simulink model "tankmodel_nonlinear_control101"  (R2025b)
settings: Solver=VariableStepAuto  StartTime=0.0  StopTime=300  RelTol=1e-3
undefined symbols (not defined in the file or in its folder): beta1rel, beta2rel, gamma1rel, gamma2rel
settings Model: Creator=barsr  LastModifiedBy=barsr
settings RTWCC: GPUComputeCapability=3.5

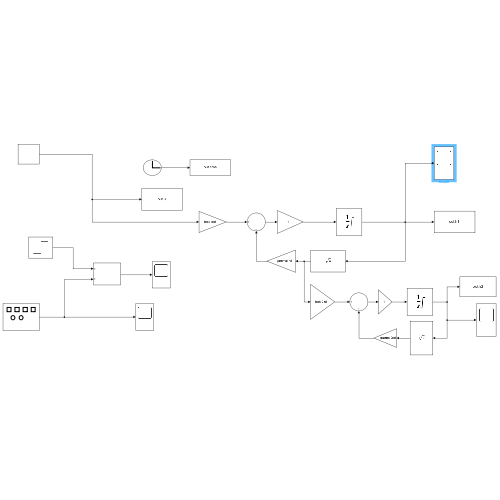
[thumbnail: Simulink's stored preview of the top-level diagram]
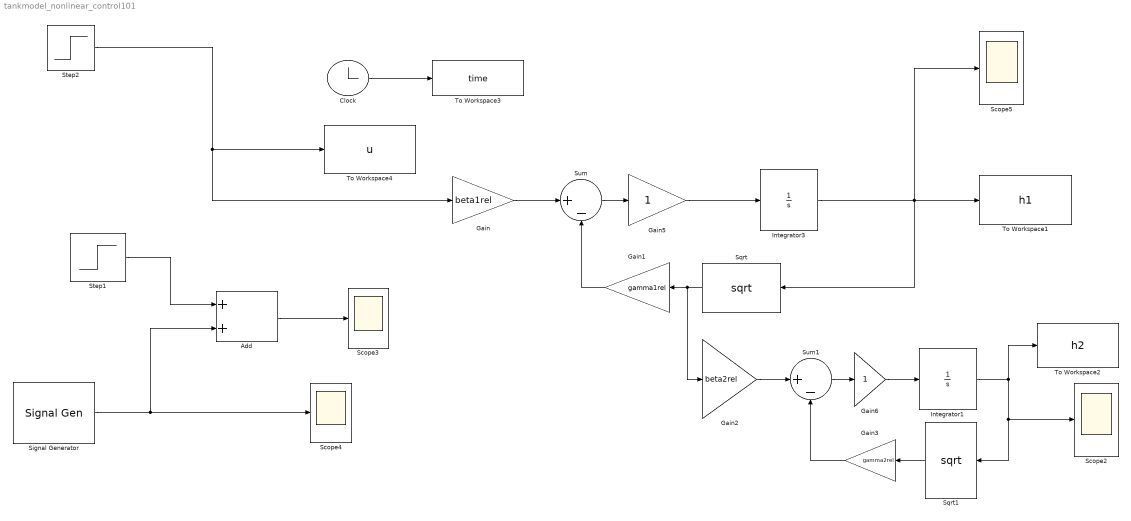
== system tankmodel_nonlinear_control101 ==
  Add : Sum
  Clock : Clock
  Gain : Gain  Gain=beta1rel
  Gain1 : Gain  Gain=gamma1rel
  Gain2 : Gain  Gain=beta2rel
  Gain3 : Gain  Gain=gamma2rel
  Gain5 : Gain
  Gain6 : Gain
  Integrator1 : Integrator  LimitOutput=on  UpperSaturationLimit=1  LowerSaturationLimit=0
  Integrator3 : Integrator  LimitOutput=on  UpperSaturationLimit=1  LowerSaturationLimit=0
  Scope{2..5} (4 alike) : Scope
      Scope2 settings: ActiveDisplayYMinimum=-0.53578092616151429  ActiveDisplayYMaximum=1.0409994632402184
      Scope3 settings: ActiveDisplayYMinimum=-1  ActiveDisplayYMaximum=1
      Scope4 settings: ActiveDisplayYMinimum=-1  ActiveDisplayYMaximum=1
      Scope5 settings: ActiveDisplayYMinimum=-0.01990953109028069  ActiveDisplayYMaximum=0.17918577981252626  DataLoggingVariableName=ScopeData2
  Signal Generator : SignalGenerator  WaveForm=square  Amplitude=0.05  Frequency=0.01  Units=rad/sec
  Sqrt : Sqrt
  Sqrt1 : Sqrt
  Step1 : Step  Time=0  After=0.25  SampleTime=0
  Step2 : Step  Time=0  After=0.25  SampleTime=0
  Sum : Sum  Inputs=|+-
  Sum1 : Sum  Inputs=|+-
  To Workspace1 : ToWorkspace  VariableName=h1  SampleTime=-1
  To Workspace2 : ToWorkspace  VariableName=h2  SampleTime=-1
  To Workspace3 : ToWorkspace  VariableName=time  SampleTime=-1
  To Workspace4 : ToWorkspace  VariableName=u  SampleTime=-1
  wires:
  Gain/1 -> Sum/1
  Sum/1 -> Gain5/1
  Sqrt/1 -> Gain2/1, Gain1/1
  Sum1/1 -> Gain6/1
  Integrator1/1 -> Sqrt1/1, Scope2/1, To Workspace2/1
  Gain6/1 -> Integrator1/1
  Sqrt1/1 -> Gain3/1
  Gain1/1 -> Sum/2
  Gain3/1 -> Sum1/2
  Gain2/1 -> Sum1/1
  Clock/1 -> To Workspace3/1
  Add/1 -> Scope3/1
  Signal Generator/1 -> Add/2, Scope4/1
  Step1/1 -> Add/1
  Gain5/1 -> Integrator3/1
  Integrator3/1 -> Scope5/1, Sqrt/1, To Workspace1/1
  Step2/1 -> Gain/1, To Workspace4/1
